simulink model "pi_test"  (R2020b)
settings: Solver=VariableStepAuto  StartTime=0.0  StopTime=10.0  RelTol=1e-3
undefined symbols (not defined in the file or in its folder): DiscIntNeverNeededParam, Pd
settings Model: Creator=SYSU-HILAB  LastModifiedBy=SYSU-HILAB

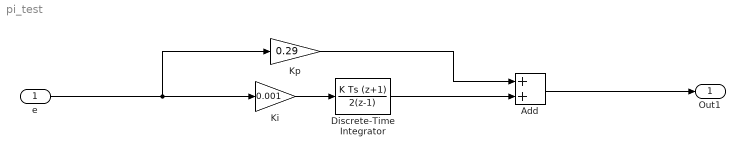
== system pi_test ==
  e : Inport
  Add : Sum
  Discrete-Time Integrator : DiscreteIntegrator  IntegratorMethod=Integration: Trapezoidal  gainval=1  SampleTime=Pd.Ts  ICPrevOutput=DiscIntNeverNeededParam  ICPrevScaledInput=DiscIntNeverNeededParam
  Ki : Gain  Gain=0.001
  Kp : Gain  Gain=0.29
  Out1 : Outport
  wires:
  Ki/1 -> Discrete-Time Integrator/1
  Kp/1 -> Add/1
  Discrete-Time Integrator/1 -> Add/2
  Add/1 -> Out1/1
  e/1 -> Kp/1, Ki/1
